simulink model "Yphase"  (R2023a)
settings: Solver=VariableStepAuto  StartTime=0.0  StopTime=(1/50)*7  FixedStep=2e-6  MaxStep=2e-6  RelTol=1e-6  EnableMultiTasking=on
libraries: spsSeriesRLCBranchLib x12, spsControlledVoltageSourceLib x4, spsCurrentMeasurementLib x4, spsACVoltageSourceLib x3, spsVoltageMeasurementLib x3, spspowerguiLib x1
settings Model: Creator=Pietro  LastModifiedBy=hp
settings SolverCC: ZeroCrossControl=DisableAll  AlgebraicLoopSolver=TrustRegion
settings DataIOCC: LimitDataPoints=on  SaveFormat=Array  SignalLoggingSaveFormat=ModelDataLogs  ReturnWorkspaceOutputs=off
settings OptimizationCC: ExpressionDepthLimit=2147483647  InitFltsAndDblsToZero=on  LifeSpan=inf
settings DebuggingCC: SaveWithParameterizedLinksMsg=none  UnderspecifiedInitializationDetection=Classic  MergeDetectMultiDrivingBlocksExec=none  SignalResolutionControl=TryResolveAllWithWarning  SolverPrmCheckMsg=warning  MultiTaskDSMMsg=warning  MultiTaskCondExecSysMsg=none  FcnCallInpInsideContextMsg=warning  UnconnectedInputMsg=warning  UnconnectedOutputMsg=warning  UnconnectedLineMsg=warning  StateNameClashWarn=warning  SFUnexpectedBacktrackingDiag=warning  SFNoUnconditionalDefaultTransitionDiag=warning  ArithmeticOperatorsInVariantConditions=warning
settings HardwareCC: ProdBitPerPointer=32  ProdBitPerSizeT=32  ProdBitPerPtrDiffT=32  ProdLargestAtomicFloat=None  ProdIntDivRoundTo=Undefined  ProdEndianess=Unspecified  ProdWordSize=32  ProdHWDeviceType=32-bit Generic
settings ModelReferenceCC: EnableRefExpFcnMdlSchedulingChecks=on  PropagateSignalLabelsOutOfModel=off
settings SFSimCC: SimUseLocalCustomCode=off  CustomCodeUndefinedFunction=UseInterfaceOnly
settings RTWCC: RTWUseLocalCustomCode=off
settings CodeAppCC: StateflowObjectComments=on
settings GRTTargetCC: TargetFcnLib=ansi_tfl_tmw.mat  TargetLangStandard=C89/C90 (ANSI)  CombineOutputUpdateFcns=off  GRTInterface=on
settings ConfigComp: CovMetricSettings=dw  CovSaveCumulativeToWorkspaceVar=on  CovSaveSingleToWorkspaceVar=on  CovExternalEMLEnable=off
settings SimscapeCC: SimscapeNormalizeSystem=off

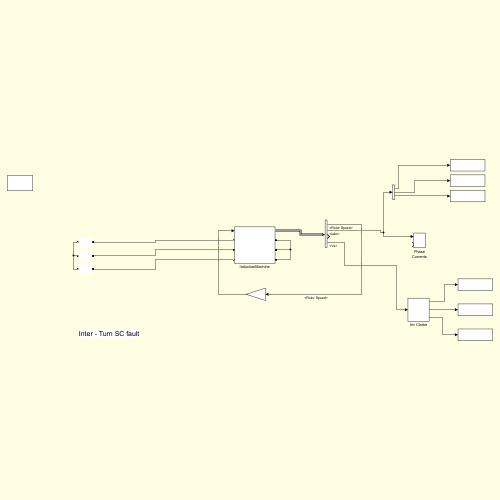
[thumbnail: Simulink's stored preview of the top-level diagram]
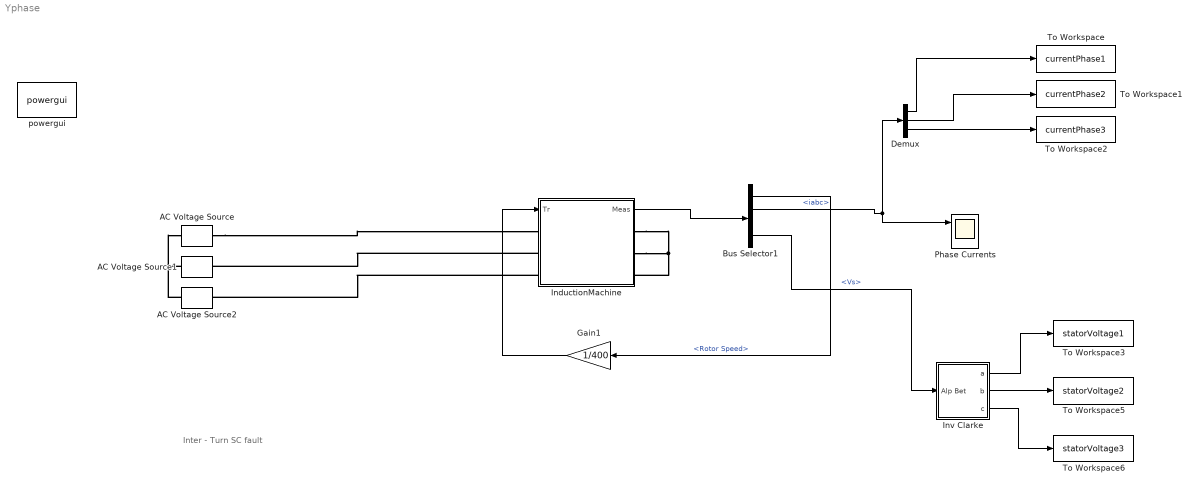
== system Yphase ==
  note: Inter - Turn SC fault
  AC Voltage Source : spsACVoltageSourceLib/AC Voltage Source  Amplitude=400/sqrt(3)  Phase=0  Frequency=50  SampleTime=-1  Measurements=None  BusType=swing  Pref=10e3  Qref=0  Qmin=-inf  Qmax=+inf
  AC Voltage Source1 : spsACVoltageSourceLib/AC Voltage Source  Amplitude=400/sqrt(3)  Phase=240  Frequency=50  SampleTime=-1  Measurements=None  BusType=swing  Pref=10e3  Qref=0  Qmin=-inf  Qmax=+inf
  AC Voltage Source2 : spsACVoltageSourceLib/AC Voltage Source  Amplitude=400/sqrt(3)  Phase=120  Frequency=50  SampleTime=-1  Measurements=None  BusType=swing  Pref=10e3  Qref=0  Qmin=-inf  Qmax=+inf
  Bus Selector1 : BusSelector  OutputSignals=Rotor Speed,iabc,Torque,Vs
  Demux : Demux  Outputs=3
  Gain1 : Gain  Gain=1/400
  InductionMachine : Subsystem  mask{Rs=1.405, Rr=1.395, Lm=0.1722, Lls=0.005839, Llr=0.005839, PP=2, J=0.0131, Kf=0.088275, Rf=143.3582}
      mask prompts: Kf "Fault Ratio"; Rf "Fault Resistance"
      mask help:
      | The initial VBR-based IM model by Pietro Tricoli,
      | Original file downloaded from:
      | https://www.mathworks.com/matlabcentral/fileexchange/53174-induction-machine-model
      mask init:
      | Lr=Llr+Lm;
      | Ls=Lls+Lm;
  Inv Clarke : Subsystem
  Phase Currents : Scope  NumInputPorts=2
  To Workspace : ToWorkspace  VariableName=currentPhase1  SampleTime=-1
  To Workspace1 : ToWorkspace  VariableName=currentPhase2  SampleTime=-1
  To Workspace2 : ToWorkspace  VariableName=currentPhase3  SampleTime=-1
  To Workspace3 : ToWorkspace  VariableName=statorVoltage1  SampleTime=-1
  To Workspace5 : ToWorkspace  VariableName=statorVoltage2  SampleTime=-1
  To Workspace6 : ToWorkspace  VariableName=statorVoltage3  SampleTime=-1
  powergui : spspowerguiLib/powergui  Priority=1  SimulationMode=Discrete  SampleTime=50e-6  frequency=60  Iterations=50  frequencyindice=0  Pbase=100e6  ErrMax=1e-4  UnitsV=kV  UnitsW=MW  buscounter=0  FunctionMessages=off  echomessages=off  EnableUseOfTLC=off  CurrentSourceSwitches=off  DisableSnubberDevices=off  DisableRonSwitches=off  DisableVfSwitches=off  DisplayEquations=off  AutomaticDiscreteSolvers=off  SolverType=Tustin  Interpol=off  ExternalGateDelay=off  methode=off  Ts=10  x0status=blocks  SPID=off  SwTol=0  HookPort=off  NonlinearTolerance=1e-4  nMaxIteration=100  ContinueOnMaxIteration=off  RestoreLinks=warning  ResistiveCurrentMeasurement=off  Frange=[0:2:500]  Ylog=off  Xlog=on  ShowGrid=off  save=off  variable=ZData  structure=0  ZoomFFT=off  StartTime=0.0  cycles=1  DisplayStyle=1  fundamental=60  FreqAxis=off  MaxFrequency=1000  frequencyindicesteady=1  RmsSteady=1  display=off
  wires:
  InductionMachine/1(Meas) -> Bus Selector1/1
  Bus Selector1/1 -> Gain1/1  "<Rotor Speed>"
  Bus Selector1/2 -> Demux/1, Phase Currents/1  "<iabc>"
  Gain1/1 -> InductionMachine/1(Tr)
  Bus Selector1/4 -> Inv Clarke/1(Alp Bet)  "<Vs>"
  Demux/1 -> To Workspace/1
  Demux/2 -> To Workspace1/1
  Demux/3 -> To Workspace2/1
  Inv Clarke/1(a) -> To Workspace3/1
  Inv Clarke/2(b) -> To Workspace5/1
  Inv Clarke/3(c) -> To Workspace6/1
  connections:
  AC Voltage Source/RConn1 -- InductionMachine/LConn1
  InductionMachine/RConn1 -- InductionMachine/RConn3 -- InductionMachine/RConn2
  InductionMachine/LConn3 -- AC Voltage Source2/RConn1
  InductionMachine/LConn2 -- AC Voltage Source1/RConn1
  AC Voltage Source2/LConn1 -- AC Voltage Source/LConn1 -- AC Voltage Source1/LConn1

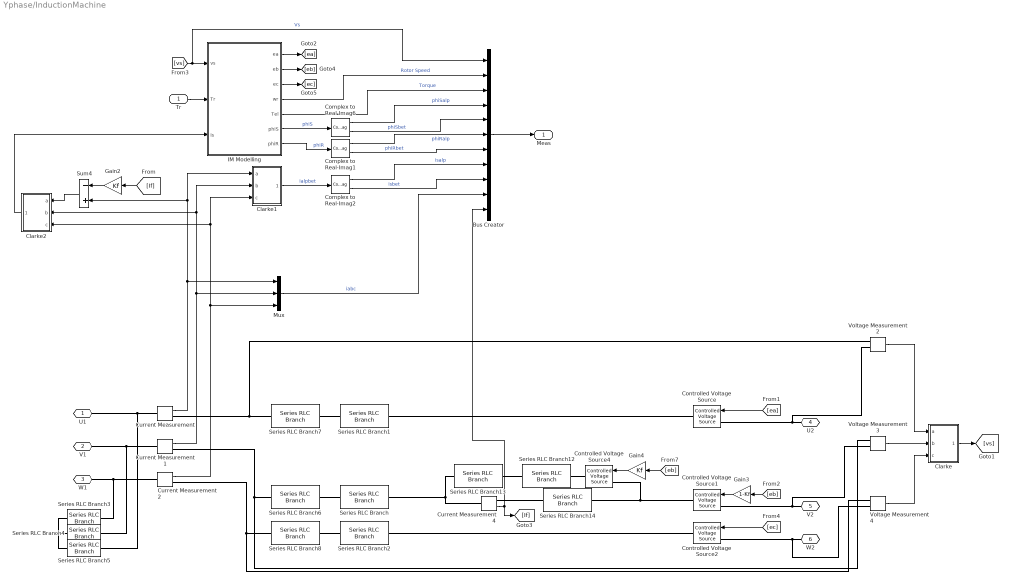
== system Yphase/InductionMachine ==
  Tr : Inport
  Bus Creator : BusCreator  Inputs=11
  Clarke : Subsystem
  Clarke1 : Subsystem
  Clarke2 : Subsystem
  Complex to Real-Imag1 : ComplexToRealImag
  Complex to Real-Imag2 : ComplexToRealImag
  Complex to Real-Imag6 : ComplexToRealImag
  Controlled Voltage Source{,1..2,4} (4 alike) : spsControlledVoltageSourceLib/Controlled Voltage Source  Initialize=on  Source_Type=AC  Amplitude=0  Phase=0  Frequency=0  Measurements=None
  Current Measurement{,1..2,4} (4 alike) : spsCurrentMeasurementLib/Current Measurement  PhasorSimulation=off  OutputType=Complex  PSBequivalent=0
  Gain2 : Gain  Gain=Kf
  Gain3 : Gain  Gain=1-Kf
  Gain4 : Gain  Gain=Kf
  IM Modelling : Subsystem
  Mux : Mux  Inputs=3
  Series RLC Branch : spsSeriesRLCBranchLib/Series RLC Branch  LConnTagsString=__new0  RConnTagsString=__new0  BranchType=L  Resistance=Rs  Inductance=Lls*(1-Kf)  SetiL0=off  InitialCurrent=0  Capacitance=1e-6  Setx0=off  InitialVoltage=0  Measurements=None
  Series RLC Branch1 : spsSeriesRLCBranchLib/Series RLC Branch  LConnTagsString=__new0  RConnTagsString=__new0  BranchType=L  Resistance=Rs  Inductance=Lls  SetiL0=on  InitialCurrent=0  Capacitance=1e-6  Setx0=off  InitialVoltage=0  Measurements=None
  Series RLC Branch12 : spsSeriesRLCBranchLib/Series RLC Branch  LConnTagsString=__new0  RConnTagsString=__new0  BranchType=L  Resistance=Rs  Inductance=Lls*Kf  SetiL0=off  InitialCurrent=0  Capacitance=1e-6  Setx0=off  InitialVoltage=0  Measurements=None
  Series RLC Branch13 : spsSeriesRLCBranchLib/Series RLC Branch  LConnTagsString=__new0  RConnTagsString=__new0  BranchType=R  Resistance=Rs*Kf  Inductance=Lls  SetiL0=off  InitialCurrent=0  Capacitance=1e-6  Setx0=off  InitialVoltage=0  Measurements=None
  Series RLC Branch14 : spsSeriesRLCBranchLib/Series RLC Branch  LConnTagsString=__new0  RConnTagsString=__new0  BranchType=R  Resistance=Rf  Inductance=Lls  SetiL0=on  InitialCurrent=0  Capacitance=1e-6  Setx0=off  InitialVoltage=0  Measurements=None
  Series RLC Branch2 : spsSeriesRLCBranchLib/Series RLC Branch  LConnTagsString=__new0  RConnTagsString=__new0  BranchType=L  Resistance=Rs  Inductance=Lls  SetiL0=on  InitialCurrent=0  Capacitance=1e-6  Setx0=off  InitialVoltage=0  Measurements=None
  Series RLC Branch3 : spsSeriesRLCBranchLib/Series RLC Branch  LConnTagsString=__new0  RConnTagsString=__new0  BranchType=R  Resistance=1e12  Inductance=Lls  SetiL0=off  InitialCurrent=0  Capacitance=1e-6  Setx0=off  InitialVoltage=0  Measurements=None
  Series RLC Branch4 : spsSeriesRLCBranchLib/Series RLC Branch  LConnTagsString=__new0  RConnTagsString=__new0  BranchType=R  Resistance=1e12  Inductance=Lls  SetiL0=off  InitialCurrent=0  Capacitance=1e-6  Setx0=off  InitialVoltage=0  Measurements=None
  Series RLC Branch5 : spsSeriesRLCBranchLib/Series RLC Branch  LConnTagsString=__new0  RConnTagsString=__new0  BranchType=R  Resistance=1e12  Inductance=Lls  SetiL0=off  InitialCurrent=0  Capacitance=1e-6  Setx0=off  InitialVoltage=0  Measurements=None
  Series RLC Branch6 : spsSeriesRLCBranchLib/Series RLC Branch  LConnTagsString=__new0  RConnTagsString=__new0  BranchType=R  Resistance=Rs*(1-Kf)  Inductance=Lls  SetiL0=off  InitialCurrent=0  Capacitance=1e-6  Setx0=off  InitialVoltage=0  Measurements=None
  Series RLC Branch7 : spsSeriesRLCBranchLib/Series RLC Branch  LConnTagsString=__new0  RConnTagsString=__new0  BranchType=R  Resistance=Rs  Inductance=Lls  SetiL0=on  InitialCurrent=0  Capacitance=1e-6  Setx0=off  InitialVoltage=0  Measurements=None
  Series RLC Branch8 : spsSeriesRLCBranchLib/Series RLC Branch  LConnTagsString=__new0  RConnTagsString=__new0  BranchType=R  Resistance=Rs  Inductance=Lls  SetiL0=on  InitialCurrent=0  Capacitance=1e-6  Setx0=off  InitialVoltage=0  Measurements=None
  Sum4 : Sum  Inputs=-+
  Voltage Measurement2 : spsVoltageMeasurementLib/Voltage Measurement  PhasorSimulation=off  OutputType=Complex  PSBequivalent=0
  Voltage Measurement3 : spsVoltageMeasurementLib/Voltage Measurement  PhasorSimulation=off  OutputType=Complex  PSBequivalent=0
  Voltage Measurement4 : spsVoltageMeasurementLib/Voltage Measurement  PhasorSimulation=off  OutputType=Complex  PSBequivalent=0
  U1 : PMIOPort  Side=Left
  V1 : PMIOPort  Port=2  Side=Left
  W1 : PMIOPort  Port=3  Side=Left
  U2 : PMIOPort  Port=4  Side=Right
  V2 : PMIOPort  Port=5  Side=Right
  W2 : PMIOPort  Port=6  Side=Right
  Meas : Outport
  wires:
  Tr/1 -> IM Modelling/2(Tr)
  Current Measurement1/1 -> Clarke2/2(b), Clarke1/2(b), Mux/2
  Current Measurement/1 -> Clarke1/1(a), Sum4/2, Mux/1
  IM Modelling/1(ea) -> [ea]
  IM Modelling/2(eb) -> [eb]
  IM Modelling/3(ec) -> [ec]
  IM Modelling/4(wr) -> Bus Creator/2  "Rotor Speed"
  [vs] -> Bus Creator/1, IM Modelling/1(vs)  "Vs"
  Voltage Measurement2/1 -> Clarke/1(a)
  Voltage Measurement3/1 -> Clarke/2(b)
  Voltage Measurement4/1 -> Clarke/3(c)
  Clarke/1(alp bet) -> [vs]
  IM Modelling/5(Tel) -> Bus Creator/3  "Torque"
  Bus Creator/1 -> Meas/1
  Complex to Real-Imag6/1 -> Bus Creator/4  "phiSalp"
  Complex to Real-Imag6/2 -> Bus Creator/5  "phiSbet"
  IM Modelling/6(phiS) -> Complex to Real-Imag6/1  "phiS"
  IM Modelling/7(phiR) -> Complex to Real-Imag1/1  "phiR"
  Complex to Real-Imag1/1 -> Bus Creator/6  "phiRalp"
  Complex to Real-Imag1/2 -> Bus Creator/7  "phiRbet"
  Clarke1/1(alp bet) -> Complex to Real-Imag2/1  "ialpbet"
  Complex to Real-Imag2/1 -> Bus Creator/8  "isalp"
  Complex to Real-Imag2/2 -> Bus Creator/9  "isbet"
  Mux/1 -> Bus Creator/10  "iabc"
  [ea] -> Controlled Voltage Source/1
  [ec] -> Controlled Voltage Source2/1
  Current Measurement2/1 -> Clarke1/3(c), Clarke2/3(c), Mux/3
  Sum4/1 -> Clarke2/1(a)
  Gain2/1 -> Sum4/1
  [If] -> Gain2/1
  Clarke2/1(alp bet) -> IM Modelling/3(Is)
  Gain3/1 -> Controlled Voltage Source1/1
  [eb] -> Gain3/1
  Current Measurement4/1 -> [If], Bus Creator/11
  Gain4/1 -> Controlled Voltage Source4/1
  [eb] -> Gain4/1
  connections:
  U1/RConn1 -- Series RLC Branch5/RConn1 -- Current Measurement/LConn1
  Current Measurement1/LConn1 -- Series RLC Branch4/RConn1 -- V1/RConn1
  Current Measurement2/LConn1 -- Series RLC Branch3/RConn1 -- W1/RConn1
  V2/RConn1 -- Voltage Measurement3/LConn2 -- Controlled Voltage Source1/LConn1
  W2/RConn1 -- Voltage Measurement4/LConn2 -- Controlled Voltage Source2/LConn1
  Controlled Voltage Source/LConn1 -- Voltage Measurement2/LConn2 -- U2/RConn1
  Series RLC Branch3/LConn1 -- Series RLC Branch4/LConn1 -- Series RLC Branch5/LConn1
  Series RLC Branch8/RConn1 -- Series RLC Branch2/LConn1
  Series RLC Branch7/RConn1 -- Series RLC Branch1/LConn1
  Series RLC Branch6/RConn1 -- Series RLC Branch/LConn1
  Voltage Measurement2/LConn1 -- Series RLC Branch7/LConn1 -- Current Measurement/RConn1
  Voltage Measurement3/LConn1 -- Current Measurement1/RConn1 -- Series RLC Branch6/LConn1
  Series RLC Branch8/LConn1 -- Current Measurement2/RConn1 -- Voltage Measurement4/LConn1
  Controlled Voltage Source2/RConn1 -- Series RLC Branch2/RConn1
  Series RLC Branch14/RConn1 -- Controlled Voltage Source1/RConn1 -- Controlled Voltage Source4/LConn1
  Current Measurement4/LConn1 -- Series RLC Branch13/LConn1 -- Series RLC Branch/RConn1
  Series RLC Branch13/RConn1 -- Series RLC Branch12/LConn1
  Current Measurement4/RConn1 -- Series RLC Branch14/LConn1
  Controlled Voltage Source4/RConn1 -- Series RLC Branch12/RConn1
  Series RLC Branch1/RConn1 -- Controlled Voltage Source/RConn1

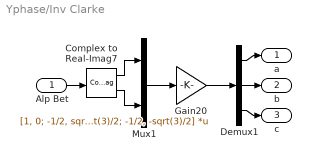
== system Yphase/Inv Clarke ==
  Alp Bet : Inport
  Complex to Real-Imag7 : ComplexToRealImag
  Demux1 : Demux  Outputs=3
  Gain20 : Gain  Gain=[1, 0; -1/2, sqrt(3)/2; -1/2, -sqrt(3)/2]  Multiplication=Matrix(K*u)
  Mux1 : Mux  Inputs=2
  a : Outport
  b : Outport  Port=2
  c : Outport  Port=3
  wires:
  Mux1/1 -> Gain20/1
  Complex to Real-Imag7/2 -> Mux1/2
  Alp Bet/1 -> Complex to Real-Imag7/1
  Demux1/2 -> b/1
  Demux1/3 -> c/1
  Gain20/1 -> Demux1/1
  Demux1/1 -> a/1
  Complex to Real-Imag7/1 -> Mux1/1

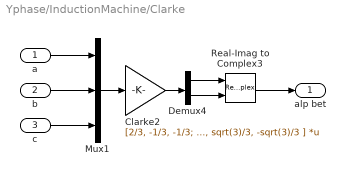
== system Yphase/InductionMachine/Clarke ==
  a : Inport
  b : Inport  Port=2
  c : Inport  Port=3
  Clarke2 : Gain  Gain=[2/3, -1/3, -1/3; 0, sqrt(3)/3, -sqrt(3)/3 ]  Multiplication=Matrix(K*u)
  Demux4 : Demux  Outputs=2
  Mux1 : Mux  Inputs=3
  Real-Imag to Complex3 : RealImagToComplex
  alp bet : Outport
  wires:
  Mux1/1 -> Clarke2/1
  Clarke2/1 -> Demux4/1
  a/1 -> Mux1/1
  Demux4/1 -> Real-Imag to Complex3/1
  Real-Imag to Complex3/1 -> alp bet/1
  Demux4/2 -> Real-Imag to Complex3/2
  c/1 -> Mux1/3
  b/1 -> Mux1/2

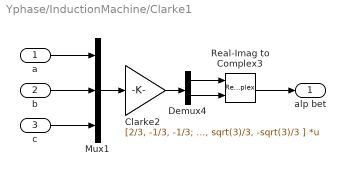
== system Yphase/InductionMachine/Clarke1 ==
  a : Inport
  b : Inport  Port=2
  c : Inport  Port=3
  Clarke2 : Gain  Gain=[2/3, -1/3, -1/3; 0, sqrt(3)/3, -sqrt(3)/3 ]  Multiplication=Matrix(K*u)
  Demux4 : Demux  Outputs=2
  Mux1 : Mux  Inputs=3
  Real-Imag to Complex3 : RealImagToComplex
  alp bet : Outport
  wires:
  Mux1/1 -> Clarke2/1
  Clarke2/1 -> Demux4/1
  a/1 -> Mux1/1
  Demux4/1 -> Real-Imag to Complex3/1
  Real-Imag to Complex3/1 -> alp bet/1
  Demux4/2 -> Real-Imag to Complex3/2
  c/1 -> Mux1/3
  b/1 -> Mux1/2

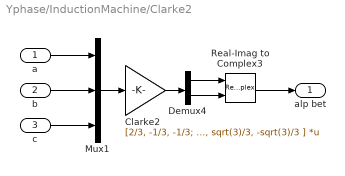
== system Yphase/InductionMachine/Clarke2 ==
  a : Inport
  b : Inport  Port=2
  c : Inport  Port=3
  Clarke2 : Gain  Gain=[2/3, -1/3, -1/3; 0, sqrt(3)/3, -sqrt(3)/3 ]  Multiplication=Matrix(K*u)
  Demux4 : Demux  Outputs=2
  Mux1 : Mux  Inputs=3
  Real-Imag to Complex3 : RealImagToComplex
  alp bet : Outport
  wires:
  b/1 -> Mux1/2
  c/1 -> Mux1/3
  Demux4/2 -> Real-Imag to Complex3/2
  Real-Imag to Complex3/1 -> alp bet/1
  Demux4/1 -> Real-Imag to Complex3/1
  a/1 -> Mux1/1
  Clarke2/1 -> Demux4/1
  Mux1/1 -> Clarke2/1

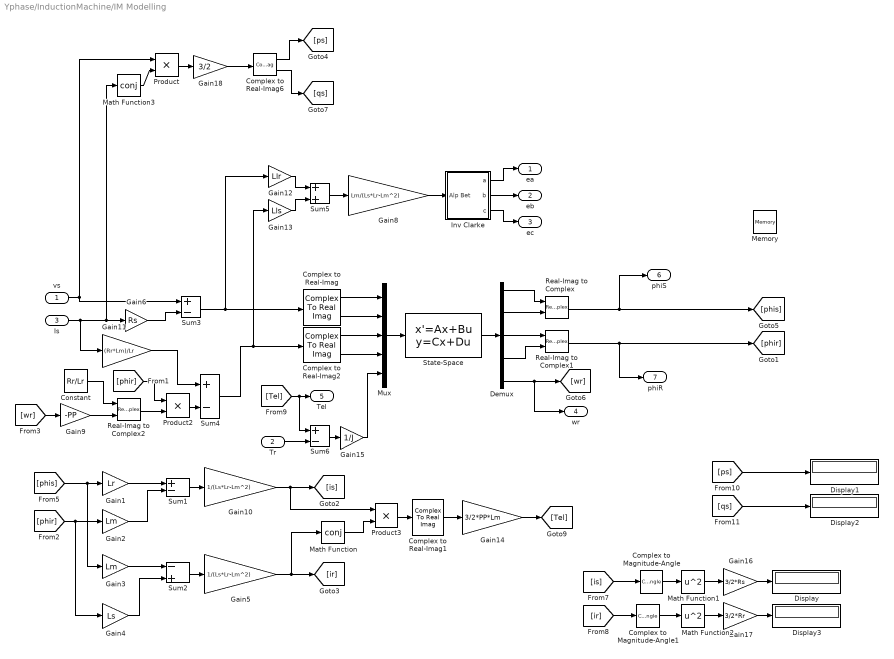
== system Yphase/InductionMachine/IM Modelling ==
  vs : Inport
  Tr : Inport  Port=2
  Is : Inport  Port=3
  Complex to Magnitude-Angle : ComplexToMagnitudeAngle  Output=Magnitude
  Complex to Magnitude-Angle1 : ComplexToMagnitudeAngle  Output=Magnitude
  Complex to Real-Imag : ComplexToRealImag
  Complex to Real-Imag1 : ComplexToRealImag  Output=Imag
  Complex to Real-Imag2 : ComplexToRealImag
  Complex to Real-Imag6 : ComplexToRealImag
  Constant : Constant  Value=Rr/Lr
  Demux : Demux  Outputs=5
  Display{,1..3} (4 alike) : Display
  Gain1 : Gain  Gain=Lr
  Gain10 : Gain  Gain=1/(Ls*Lr-Lm^2)
  Gain11 : Gain  Gain=(Rr*Lm)/Lr
  Gain12 : Gain  Gain=Llr
  Gain13 : Gain  Gain=Lls
  Gain14 : Gain  Gain=3/2*PP*Lm
  Gain15 : Gain  Gain=1/J
  Gain16 : Gain  Gain=3/2*Rs
  Gain17 : Gain  Gain=3/2*Rr
  Gain18 : Gain  Gain=3/2
  Gain2 : Gain  Gain=Lm
  Gain3 : Gain  Gain=Lm
  Gain4 : Gain  Gain=Ls
  Gain5 : Gain  Gain=1/(Ls*Lr-Lm^2)
  Gain6 : Gain  Gain=Rs
  Gain8 : Gain  Gain=Lm/(Ls*Lr-Lm^2)
  Gain9 : Gain  Gain=-PP
  Inv Clarke : Subsystem
  Math Function : Math  Operator=conj  SignedPower=on
  Math Function1 : Math  Operator=square  SignedPower=on
  Math Function2 : Math  Operator=square  SignedPower=on
  Math Function3 : Math  Operator=conj  SignedPower=on
  Memory : Memory  InheritSampleTime=on
  Mux : Mux  Inputs=5
  Product : Product  RndMeth=Zero
  Product2 : Product  RndMeth=Zero
  Product3 : Product  RndMeth=Zero
  Real-Imag to Complex : RealImagToComplex
  Real-Imag to Complex1 : RealImagToComplex
  Real-Imag to Complex2 : RealImagToComplex
  State-Space : StateSpace  A=[0,0,0,0,0; 0,0,0,0,0; 0,0,0,0,0; 0,0,0,0,0; 0,0,0,0,0]  B=[1,0,0,0,0; 0,1,0,0,0; 0,0,1,0,0; 0,0,0,1,0; 0,0,0,0,1]  C=[1,0,0,0,0; 0,1,0,0,0; 0,0,1,0,0; 0,0,0,1,0; 0,0,0,0,1]  D=[0,0,0,0,0; 0,0,0,0,0; 0,0,0,0,0; 0,0,0,0,0; 0,0,0,0,0]  InitialCondition=[0,0,0,0,0]
  Sum{1,3..4,6} (4 alike) : Sum  Inputs=+-
  Sum2 : Sum  Inputs=-+
  Sum5 : Sum
  ea : Outport
  eb : Outport  Port=2
  ec : Outport  Port=3
  wr : Outport  Port=4
  Tel : Outport  Port=5
  phiS : Outport  Port=6
  phiR : Outport  Port=7
  wires:
  Demux/1 -> Real-Imag to Complex/1
  Demux/2 -> Real-Imag to Complex/2
  Complex to Real-Imag/1 -> Mux/1
  Complex to Real-Imag/2 -> Mux/2
  Gain14/1 -> [Tel]
  Sum6/1 -> Gain15/1
  [Tel] -> Sum6/1, Tel/1
  Tr/1 -> Sum6/2
  Demux/5 -> wr/1, [wr]
  Demux/3 -> Real-Imag to Complex1/1
  Demux/4 -> Real-Imag to Complex1/2
  Gain15/1 -> Mux/5
  [phis] -> Gain1/1, Gain3/1
  Gain1/1 -> Sum1/1
  Gain2/1 -> Sum1/2
  [phir] -> Gain4/1, Gain2/1
  Sum1/1 -> Gain10/1
  Gain3/1 -> Sum2/1
  Gain4/1 -> Sum2/2
  Sum2/1 -> Gain5/1
  Complex to Real-Imag2/1 -> Mux/3
  Complex to Real-Imag2/2 -> Mux/4
  Gain5/1 -> Math Function/1, [ir]
  Complex to Real-Imag1/1 -> Gain14/1
  Product3/1 -> Complex to Real-Imag1/1
  Math Function/1 -> Product3/2
  Is/1 -> Gain11/1, Math Function3/1, Gain6/1
  vs/1 -> Product/1, Sum3/1
  Sum5/1 -> Gain8/1
  Gain13/1 -> Sum5/2
  Gain12/1 -> Sum5/1
  [is] -> Complex to Magnitude-Angle/1
  Complex to Magnitude-Angle/1 -> Math Function1/1
  Math Function1/1 -> Gain16/1
  Gain16/1 -> Display/1
  [ir] -> Complex to Magnitude-Angle1/1
  Complex to Magnitude-Angle1/1 -> Math Function2/1
  Math Function2/1 -> Gain17/1
  Gain17/1 -> Display3/1
  [ps] -> Display1/1
  [qs] -> Display2/1
  Product/1 -> Gain18/1
  Math Function3/1 -> Product/2
  Gain18/1 -> Complex to Real-Imag6/1
  Complex to Real-Imag6/1 -> [ps]
  Complex to Real-Imag6/2 -> [qs]
  Mux/1 -> State-Space/1
  Gain8/1 -> Inv Clarke/1(Alp Bet)
  Inv Clarke/3(c) -> ec/1
  Inv Clarke/1(a) -> ea/1
  Inv Clarke/2(b) -> eb/1
  State-Space/1 -> Demux/1
  Gain10/1 -> Product3/1, [is]
  [wr] -> Gain9/1
  Gain9/1 -> Real-Imag to Complex2/2
  Constant/1 -> Real-Imag to Complex2/1
  Real-Imag to Complex2/1 -> Product2/2
  [phir] -> Product2/1
  Product2/1 -> Sum4/2
  Gain11/1 -> Sum4/1
  Sum4/1 -> Gain13/1, Complex to Real-Imag2/1
  Real-Imag to Complex/1 -> [phis], phiS/1
  Real-Imag to Complex1/1 -> [phir], phiR/1
  Gain6/1 -> Sum3/2
  Sum3/1 -> Gain12/1, Complex to Real-Imag/1

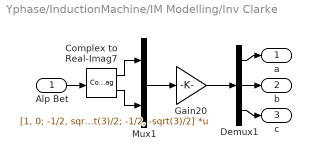
== system Yphase/InductionMachine/IM Modelling/Inv Clarke ==
  Alp Bet : Inport
  Complex to Real-Imag7 : ComplexToRealImag
  Demux1 : Demux  Outputs=3
  Gain20 : Gain  Gain=[1, 0; -1/2, sqrt(3)/2; -1/2, -sqrt(3)/2]  Multiplication=Matrix(K*u)
  Mux1 : Mux  Inputs=2
  a : Outport
  b : Outport  Port=2
  c : Outport  Port=3
  wires:
  Mux1/1 -> Gain20/1
  Complex to Real-Imag7/2 -> Mux1/2
  Alp Bet/1 -> Complex to Real-Imag7/1
  Demux1/2 -> b/1
  Demux1/3 -> c/1
  Gain20/1 -> Demux1/1
  Demux1/1 -> a/1
  Complex to Real-Imag7/1 -> Mux1/1
